simulink model "flexpwm_ctu_adc_center"  (Simulink 8.1)
settings: Solver=FixedStepDiscrete  StartTime=0.0  StopTime=10.0  FixedStep=0.2  RelTol=1e-3
undefined symbols (not defined in the file or in its folder): A10, A14, AN0, AN12, AN8, B, B13, D, D11, K4, L3, P3, PA11, PA12, PB10, PB13, PB7, PC14, PC7, PD6, PE5, R10, R5, R8, T5
libraries: rappid_564xl_ec_toolbox x10
settings Model: Creator=evarshavskaya  LastModifiedBy=evarshavskaya
settings DataIOCC: ExternalInput=off  InitialState=off  SaveOutput=off  SignalLogging=off  SaveTime=off
settings OptimizationCC: InlineParams=on  OptimizeModelRefInitCode=on  LifeSpan=1
settings DebuggingCC: InheritedTsInSrcMsg=none  SingleTaskRateTransMsg=error  UnconnectedInputMsg=error  UnconnectedOutputMsg=error  UnconnectedLineMsg=error  UnknownTsInhSupMsg=error
settings HardwareCC: ProdLargestAtomicInteger=Long  ProdLargestAtomicFloat=Double  ProdIntDivRoundTo=Zero  ProdEndianess=BigEndian  ProdHWDeviceType=Freescale->32-bit PowerPC
settings RTWCC: SystemTargetFile=rappid564xl.tlc  MakeCommand=rappid_564xl_make_rtw  TemplateMakefile=rappid_564xl_default_tmf  PostCodeGenCommand=rappid_analyzegencode(buildInfo)  Description=RAppID Toolbox MPC564xL Code Generation Target (rappid)  ProcessScript=rappid564xl_make_rtw_hook
settings CodeAppCC: IgnoreCustomStorageClasses=off  CustomSymbolStrType=$N$R$M  InternalIdentifier=Classic
settings STFCustomTargetCC: CodeReplacementLibrary=ANSI_C  ModelReferenceCompliant=off  CombineOutputUpdateFcns=on  SuppressErrorStatus=on  ERTCustomFileBanners=on  SupportContinuousTime=off  SupportNonInlinedSFcns=off  MATLABClassNameForMDSCustomization=Simulink.SoftwareTarget.ERTCustomization  GRTInterface=off  SystemTargetFile=rappid564xl.tlc
settings ERTTargetCC: CodeReplacementLibrary=ANSI_C  MultiwordLength=2048  ModelReferenceCompliant=off  ParMdlRefBuildCompliant=off  CompOptLevelCompliant=off  ConcurrentExecutionCompliant=off  SuppressErrorStatus=on  ERTFirstTimeCompliant=off  ModelStepFunctionPrototypeControlCompliant=off  CPPClassGenCompliant=off  ExtModeMexFile=noextcomm  InlinedParameterPlacement=NonHierarchical  ERTCustomFileTemplate=example_file_process.tlc  ConvertIfToSwitch=off  SuppressUnreachableDefaultCases=off

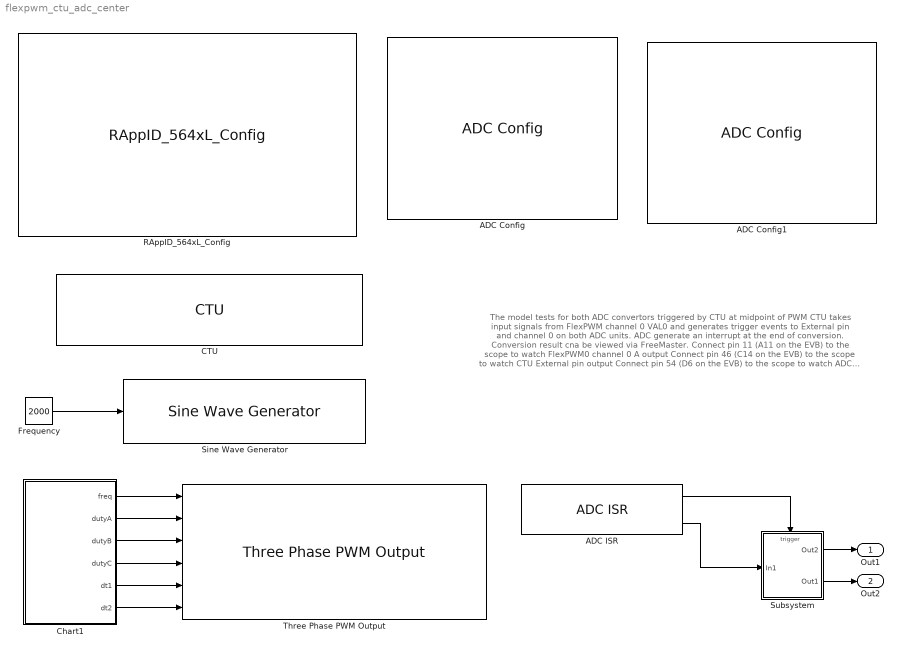
== system flexpwm_ctu_adc_center ==
  note: The model tests for both ADC convertors triggered by CTU at midpoint of PWM
      |
      | CTU takes input signals from FlexPWM channel 0 VAL0 and generates trigger events to External pin and channel 0 on both ADC units.
      | ADC generate an interrupt at the end of conversion. Conversion result cna be viewed via FreeMaster.
      |
      | Connect pin 11 (A11 on the EVB) to the scope to watch FlexPWM0 channel 0 A output
      | Connect pin 46 (C14 on the EVB) to the scope to watch CTU External pin output
      | Connect pin 54 (D6 on the EVB) to the scope to watch ADC End of CTU conversion interrupt
      | Connect pin 23 (B7 on the EVB) to the source of the signal (SWG output pin D7 as example) to provide data to the ADC0 Channel 0.
      | Connect pin 29 (B13 on the EVB) to the source of the signal (SWG output pin D7 as example) to provide data to the ADC1 Channel 0.
  ADC Config : rappid_564xl_ec_toolbox/MPC564xL/Motor Control Blocks/ADC Config  adc_unit=0  adc_ctu=on  adc_owr=on  adc_wls=Left  adc_clk=on  adc_ack=on  adc_ctr0_inp=off  adc_ctr0_shft=10 - Avin = 0  adc_ctr0_cmp=01  adc_ctr0_samp=4  adc_ctr1_inp=off  adc_ctr1_cmp=01  adc_ctr1_samp=1  adc_ctr1_tsens=PTAT  adc_pscr_preval=V0  adc_pscr_preconv=off
  ADC Config1 : rappid_564xl_ec_toolbox/MPC564xL/Motor Control Blocks/ADC Config  adc_unit=1  adc_ctu=on  adc_owr=on  adc_wls=Left  adc_clk=on  adc_ack=on  adc_ctr0_inp=off  adc_ctr0_shft=10 - Avin = 0  adc_ctr0_cmp=01  adc_ctr0_samp=4  adc_ctr1_inp=off  adc_ctr1_cmp=01  adc_ctr1_samp=1  adc_ctr1_tsens=PTAT  adc_pscr_preval=V0  adc_pscr_preconv=off
  ADC ISR : rappid_564xl_ec_toolbox/MPC564xL/Motor Control Blocks/ADC ISR  adc_unit=0  adc_isr_pri=15  adc_isr_ech=off  adc_isr_eoc=off  adc_isr_jech=off  adc_isr_jeoc=off  adc_isr_eoctu=on
  CTU : rappid_564xl_ec_toolbox/MPC564xL/Motor Control Blocks/CTU  ModeEdit=Triggered  Mode=0  MRSedit=PWM reload Rising edge  MRS=0  MaxDelay=1000  ExtTgrPin_0="46  : PC14 : [ 103 ] : [ E15 ]"  ExtInPin_0=None  extTgrPcr=46  extInPcr=255  InputSelection=12  PWM_REL=Disabled  PWM_ODD_0=Rising and Falling  PWM_ODD_1=Disabled  PWM_ODD_2=Disabled  PWM_ODD_3=Disabled  PWM_EVEN_0=Disabled  PWM_EVEN_1=Disabled  PWM_EVEN_2=Disabled  PWM_EVEN_3=Disabled  RPWM_0=Disabled  RPWM_1=Disabled  RPWM_2=Disabled  RPWM_3=Disabled  eTimer_0=Disabled  eTimer_1=Disabled  External=Disabled  TriggerOutput_1=97  TriggerOutput_2=0  ADC_CmdIndex_1=0  ADC_CmdIndex_2=0  ADC_Cmd_1=57344  ADC_Cmd_2=16384  ADC_Cmd_3=0  ADC_Cmd_4=0  ADC_Cmd_5=0  ADC_Cmd_6=0  ADC_Cmd_7=0  ADC_Cmd_8=0  ADC_Cmd_9=0  ADC_Cmd_10=0  ADC_Cmd_11=0  ADC_Cmd_12=0  ADC_Cmd_13=0  ADC_Cmd_14=0  ADC_Cmd_15=0  ADC_Cmd_16=0  ADC_Cmd_17=0  ADC_Cmd_18=0  ADC_Cmd_19=0  ADC_Cmd_20=0  ADC_Cmd_21=0  ADC_Cmd_22=0  ADC_Cmd_23=0  ADC_Cmd_24=0  T0_E=on  T0_ETE=on  T0_T0E=off  T0_T1E=off  T0_T2E=off  T0_ADCE=on  T0_Delay=0  T1_E=off  T1_ETE=off  T1_T0E=off  T1_T1E=off  T1_T2E=off  T1_ADCE=off  T1_Delay=100  T2_E=off  T2_ETE=off  T2_T0E=off  T2_T1E=off  T2_T2E=off  T2_ADCE=off  T2_Delay=0  T3_E=off  T3_ETE=off  T3_T0E=off  T3_T1E=off  T3_T2E=off  T3_ADCE=off  T3_Delay=0  T4_E=off  T4_ETE=off  T4_T0E=off  T4_T1E=off  T4_T2E=off  T4_ADCE=off  T4_Delay=0  T5_E=off  T5_ETE=off  T5_T0E=off  T5_T1E=off  T5_T2E=off  T5_ADCE=off  T5_Delay=0  T6_E=off  T6_ETE=off  T6_T0E=off  T6_T1E=off  T6_T2E=off  T6_ADCE=off  T6_Delay=0  T7_E=off  T7_ETE=off  T7_T0E=off  T7_T1E=off  T7_T2E=off  T7_ADCE=off  T7_Delay=0  T_delay=0  ADC_Cmd=0  T0_ADC_num=1  T0_ADC_nlist=1  T1_ADC_num=0  T1_ADC_nlist=no commands  T2_ADC_num=0  T2_ADC_nlist=no commands  T3_ADC_num=0  T3_ADC_nlist=no commands  T4_ADC_num=0  T4_ADC_nlist=no commands  T5_ADC_num=0  T5_ADC_nlist=no commands  T6_ADC_num=0  T6_ADC_nlist=no commands  T7_ADC_num=0  T7_ADC_nlist=no commands  ADC_CMS_1=Dual-conversion mode  ADC_CIR_1=Enabled  ADC_FIFO_1=0  ADC_CHA_1=0  ADC_CHB_1=0  ADC_CMS_2=Single-conversion mode: ADC unit A  ADC_CIR_2=Enabled  ADC_FIFO_2=0  ADC_CHA_2=0  ADC_CHB_2=0  ADC_CMS_3=Single-conversion mode: ADC unit A  ADC_CIR_3=Disabled  ADC_FIFO_3=0  ADC_CHA_3=0  ADC_CHB_3=0  ADC_CMS_4=Single-conversion mode: ADC unit A  ADC_CIR_4=Disabled  ADC_FIFO_4=0  ADC_CHA_4=0  ADC_CHB_4=0  ADC_CMS_5=Single-conversion mode: ADC unit A  ADC_CIR_5=Disabled  ADC_FIFO_5=0  ADC_CHA_5=0  ADC_CHB_5=0  ADC_CMS_6=Single-conversion mode: ADC unit A  ADC_CIR_6=Disabled  ADC_FIFO_6=0  ADC_CHA_6=0  ADC_CHB_6=0  ADC_CMS_7=Single-conversion mode: ADC unit A  ADC_CIR_7=Disabled  ADC_FIFO_7=0  ADC_CHA_7=0  ADC_CHB_7=0  ADC_CMS_8=Single-conversion mode: ADC unit A  ADC_CIR_8=Disabled  ADC_FIFO_8=0  ADC_CHA_8=0  ADC_CHB_8=0  ADC_CMS_9=Single-conversion mode: ADC unit A  ADC_CIR_9=Disabled  ADC_FIFO_9=0  ADC_CHA_9=0  ADC_CHB_9=0  ADC_CMS_10=Single-conversion mode: ADC unit A  ADC_CIR_10=Disabled  ADC_FIFO_10=0  ADC_CHA_10=0  ADC_CHB_10=0  ADC_CMS_11=Single-conversion mode: ADC unit A  ADC_CIR_11=Disabled  ADC_FIFO_11=0  ADC_CHA_11=0  ADC_CHB_11=0  ADC_CMS_12=Single-conversion mode: ADC unit A  ADC_CIR_12=Disabled  ADC_FIFO_12=0  ADC_CHA_12=0  ADC_CHB_12=0  ADC_CMS_13=Single-conversion mode: ADC unit A  ADC_CIR_13=Disabled  ADC_FIFO_13=0  ADC_CHA_13=0  ADC_CHB_13=0  ADC_CMS_14=Single-conversion mode: ADC unit A  ADC_CIR_14=Disabled  ADC_FIFO_14=0  ADC_CHA_14=0  ADC_CHB_14=0  ADC_CMS_15=Single-conversion mode: ADC unit A  ADC_CIR_15=Disabled  ADC_FIFO_15=0  ADC_CHA_15=0  ADC_CHB_15=0  ADC_CMS_16=Single-conversion mode: ADC unit A  ADC_CIR_16=Disabled  ADC_FIFO_16=0  ADC_CHA_16=0  ADC_CHB_16=0  ADC_CMS_17=Single-conversion mode: ADC unit A  ADC_CIR_17=Disabled  ADC_FIFO_17=0  ADC_CHA_17=0  ADC_CHB_17=0  ADC_CMS_18=Single-conversion mode: ADC unit A  ADC_CIR_18=Disabled  ADC_FIFO_18=0  ADC_CHA_18=0  ADC_CHB_18=0  ADC_CMS_19=Single-conversion mode: ADC unit A  ADC_CIR_19=Disabled  ADC_FIFO_19=0  ADC_CHA_19=0  ADC_CHB_19=0  ADC_CMS_20=Single-conversion mode: ADC unit A  ADC_CIR_20=Disabled  ADC_FIFO_20=0  ADC_CHA_20=0  ADC_CHB_20=0  ADC_CMS_21=Single-conversion mode: ADC unit A  ADC_CIR_21=Disabled  ADC_FIFO_21=0  ADC_CHA_21=0  ADC_CHB_21=0  ADC_CMS_22=Single-conversion mode: ADC unit A  ADC_CIR_22=Disabled  ADC_FIFO_22=0  ADC_CHA_22=0  ADC_CHB_22=0  ADC_CMS_23=Single-conversion mode: ADC unit A  ADC_CIR_23=Disabled  ADC_FIFO_23=0  ADC_CHA_23=0  ADC_CHB_23=0  ADC_CMS_24=Single-conversion mode: ADC unit A  ADC_CIR_24=Disabled  ADC_FIFO_24=0  ADC_CHA_24=0  ADC_CHB_24=0  dst=|  T0_cmdNum=0  T0_ADC_CMS_1=Dual-conversion mode  T0_ADC_CIR_1=Enabled  T0_ADC_FIFO_1=0  T0_ADC_CHA_1=0  T0_ADC_CHB_1=0  T0_ADC_CMS_2=Dual-conversion mode  T0_ADC_CIR_2=Enabled  T0_ADC_FIFO_2=0  T0_ADC_CHA_2=0  T0_ADC_CHB_2=0  T0_ADC_CMS_3=Single-conversion mode: ADC unit A  T0_ADC_CIR_3=Disabled  T0_ADC_FIFO_3=0  T0_ADC_CHA_3=0  T0_ADC_CHB_3=0  T1_cmdNum=1  T1_ADC_CMS_1=Single-conversion mode: ADC unit A  T1_ADC_CIR_1=Disabled  T1_ADC_FIFO_1=0  T1_ADC_CHA_1=3  T1_ADC_CHB_1=0  T1_ADC_CMS_2=Single-conversion mode: ADC unit A  T1_ADC_CIR_2=Disabled  T1_ADC_FIFO_2=0  T1_ADC_CHA_2=0  T1_ADC_CHB_2=0  T1_ADC_CMS_3=Single-conversion mode: ADC unit A  T1_ADC_CIR_3=Disabled  T1_ADC_FIFO_3=0  T1_ADC_CHA_3=0  T1_ADC_CHB_3=0  ver=2
      | Triggered mode
      |       Input selection: 00000000 00000000 00000000 00001100
      | Trigger Output 0-3: 00000000 00000000 00000000 01100001
      | Trigger Output 4-7: 00000000 00000000 00000000 00000000
      | ADC command list size: 1
  Chart1 : Stateflow chart  TreatAsAtomicUnit=on
  Frequency : Constant  Value=2000  OutDataTypeStr=uint16
  RAppID_564xL_Config : rappid_564xl_ec_toolbox/MPC564xL/RAppID_564xL_Config  SystemClock=120  XTAL=40  MC_clock_60=12  MC_clock_80=16  MC_clock_120=10  SWG_clock_60=20  SWG_clock_80=13.334  SWG_clock_120=20  Compiler=CodeWarrior  MemTarget=RAM  Part=MPC5643L  Package=144 LQFP  global_int_priority=10  base_tick_priority=14  sys_task_supress=off  exception_handlers=off  stored_mdl_name=flexpwm_ctu_adc_center  freemaster_interface=Oops  freemaster_rx_pin="LINFlex_0 Rx Pin 116 : \"PB[3]\""  freemaster_tx_pin="LINFlex_0 Tx Pin 114 : \"PB[2]\""  freemaster_interface_1=Serial 0  freemaster_enable=on  freemaster_rate=57600  freemaster_tx0_pin=18 : B[2] : 114 : A14  freemaster_rx0_pin=19 : B[3] : 116 : B13  freemaster_tx1_pin=57 : D[9] : 26 : L3  freemaster_rx1_pin=29 : B[13] : 60 : R10  freemaster_can_channel=1CH  freemater_can_speed=500K  freemaster_can_msgig=0x7AA  ccp_interface=None  ccp_enable=off  ccp_can_channel=CH1 (MB 0 - 1)  ccp_can_speed=500K  ccp_can_cro_id=256  ccp_can_dto_id=257  ccp_dev_id=RappID  ccp_dev_addr=0  ccp_odt=3  ccp_daq=3  pil_enable=off  pil_bam=on  comport=1  pil_rate=57600  bam_password_def=on  bam_password=0xFEEDFACECAFEBEEF  bam_sa_cs=off  bam_start_address=0x0  bam_code_size=0x7000  cons_dspi=on  cons_can=on  cons_adc=on  cons_pwm=on  cons_ctu=on  cons_swg=on  cons_eTimer=on  cons_fm=on
  Sine Wave Generator : rappid_564xl_ec_toolbox/MPC564xL/Motor Control Blocks/Sine Wave Generator  amplitude=2.264  frequency=2000  IOAMPL=15
  Subsystem : Subsystem
      settings: RTWSystemCode=Nonreusable function
  Three Phase PWM Output : rappid_564xl_ec_toolbox/MPC564xL/Motor Control Blocks/Three Phase PWM Output  pwmModule=0  pwmMod=0  SubModule=0 1 2  subMod=0  InitFreq=10000  resolution=1 %  resValue=1  InitDutyA=70  InitDutyB=50  InitDutyC=30  DeadTime=50  dt=IPBus clock cycles  deadtime_mks=0  DebugSw=off  debug_mode=0  pin_A0="11  : PA11 : [ 120 ] : [ D11 ]"  pin_B0=None  pin_A1="39  : PC7  : [ 15 ] : [ K4 ]"  pin_B1=None  pin_A2="12  : PA12 : [ 122 ] : [ A10 ]"  pin_B2=None  pin_A3=None  pin_B3=None  pin1_A0=None  pin1_B0=None  pin1_A1=None  pin1_B1=None  pin1_A2=None  pin1_B2=None  pin1_A3=None  pin1_B3=None  pcrNum=0  polA0=off  polB0=off  polA1=off  polB1=off  polA2=off  polB2=off  polA3=off  polB3=off  octrl=0  outVal_A0=on  outVal_A1=off  outVal_A2=off  outVal_A3=off  outVal_B0=off  outVal_B1=off  outVal_B2=off  outVal_B3=off  outVal_C0=off  outVal_C1=off  outVal_C2=off  outVal_C3=off  outTrig=0
  Out1 : Outport
  Out2 : Outport  Port=2
  wires:
  ADC ISR/1 -> Subsystem/Trigger
  Subsystem/1(Out2) -> Out1/1
  ADC ISR/2 -> Subsystem/1(In1)
  Subsystem/2(Out1) -> Out2/1
  Chart1/1(freq) -> Three Phase PWM Output/1
  Chart1/2(dutyA) -> Three Phase PWM Output/2
  Chart1/3(dutyB) -> Three Phase PWM Output/3
  Chart1/4(dutyC) -> Three Phase PWM Output/4
  Chart1/5(dt1) -> Three Phase PWM Output/5
  Chart1/6(dt2) -> Three Phase PWM Output/6
  Frequency/1 -> Sine Wave Generator/1

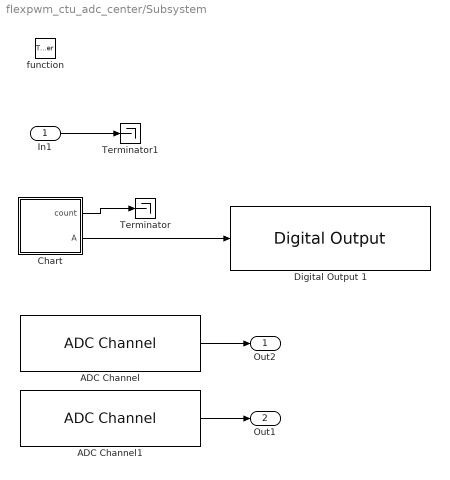
== system flexpwm_ctu_adc_center/Subsystem ==
  In1 : Inport
  function : TriggerPort  TriggerType=function-call
  ADC Channel : rappid_564xl_ec_toolbox/MPC564xL/Motor Control Blocks/ADC Channel  adc_unit=0  adc_chan0=older  adc_chan0_v2=23 : PB7 : [43] : [R5] : AN0  adc_chan1=older  adc_chan1_v2=26 : PB10 : [53] : [R8] : AN12  simulate=off  interrupt=on  adc_mode=Normal  adc_presample=off
  ADC Channel1 : rappid_564xl_ec_toolbox/MPC564xL/Motor Control Blocks/ADC Channel  adc_unit=1  adc_chan0=older  adc_chan0_v2=69 : PE5 : [44] : [T5] : AN8  adc_chan1=older  adc_chan1_v2=29 : PB13 : [60] : [R10] : AN0  simulate=off  interrupt=off  adc_mode=Normal  adc_presample=off
  Chart : Stateflow chart  TreatAsAtomicUnit=on
  Digital Output 1 : rappid_564xl_ec_toolbox/MPC564xL/General Purpose Blocks/Digital Output   gpio_outputs="54  : PD6  : [ 34 ] : [ P3 ]"  pinNum=[ 34 ]  pcrNum=54
  Terminator : Terminator
  Terminator1 : Terminator
  Out2 : Outport
  Out1 : Outport  Port=2
  wires:
  ADC Channel/1 -> Out2/1
  Chart/2(A) -> Digital Output 1/1
  Chart/1(count) -> Terminator/1
  In1/1 -> Terminator1/1
  ADC Channel1/1 -> Out1/1

== stateflow chart Subsystem/Chart ==
  state A
  state A1
  (default) -> A : {count =0;}
  A -> A1
  A1 -> A : { count = count + 1;}
  data: count output double; A output boolean

== stateflow chart Chart1 ==
  settings: executeAtInitialization=1
  state A
    en:
    freq =10000;
    dutyA=70;
    dutyB=50;
    dutyC=30;
    dt1=50;
    dt2=50;
    du:
    cntr=cntr+1;
  state A1
    en:
    freq =10000;
    dutyA=30;
    dutyB=70;
    dutyC=50;
    dt1=50;
    dt2=50;
    du:
    cntr=cntr+1;
  state A2
    en:
    freq =10000;
    dutyA=50;
    dutyB=30;
    dutyC=7;
    dt1=50;
    dt2=50;
    du:
    cntr=cntr+1;
    ex:
    cntr = 0;
  (default) -> A : {cntr=0;}
  A2 -> A : [cntr > 30]
  A -> A1 : [cntr > 10]
  A1 -> A2 : [cntr > 20]
  data: cntr local uint32 =0; freq output uint32; dutyA output uint32; dutyB output uint32; dutyC output uint32; dt1 output uint32; dt2 output uint32
